simulink model "AUV_Model"  (R2023a)
settings: Solver=VariableStepAuto  StartTime=0.0  StopTime=300  FixedStep=0.5  RelTol=1e-3
InitFcn:
  | mdlWks = get_param(gcs,'ModelWorkspace');
  | a = getVariable(mdlWks,'a');
  | b = getVariable(mdlWks,'b');
  | c = getVariable(mdlWks,'c');
StopFcn:
  | figure(2)
  | plot3(Position_Data(1,1),Position_Data(1,2),Position_Data(1,3),'r*')
  | hold on
  | plot3(Position_Data(:,1),Position_Data(:,2),Position_Data(:,3));
  | plot3(Position_Data(end,1),Position_Data(end,2),Position_Data(end,3),'g*');
  | grid on
  | legend('Start Point','Trajectory','End Point')
model workspace (MAT data in the model file):
  a = 0
  b = 1
  c = 1
undefined symbols (not defined in the file or in its folder): sigbuilder_block
libraries: sharedtransform x6, vrlib x6, dspfdesign x6, sim3dlib x3, slpidlib x3, simulink x2, shared6dof x1, aerolibasang x1, aerolibnav x1, sim3dphyssensorlib x1
(part 2 of 2)

== system AUV_Model/Plant and Environment Model/Propulsion Forces & Moments/Force and moments due to Thrust/Thrust to Propulsion  ==
  Thrust Inputs : Inport
  Demux : Demux  Outputs=5
  Moment computation : Subsystem
  Sum : Sum  Inputs=+++++
  Thrust Transformation : Subsystem
  Propulsion Force : Outport  VectorParamsAs1DForOutWhenUnconnected=off
  Propulsion Moment : Outport  Port=2  VectorParamsAs1DForOutWhenUnconnected=off
  wires:
  Demux/5 -> Moment computation/5(Pz)
  Demux/4 -> Moment computation/4(Py2)
  Demux/3 -> Moment computation/3(Py1)
  Demux/2 -> Moment computation/2(Px2)
  Demux/1 -> Moment computation/1(Px1)
  Thrust Transformation/3(Thrust Py1) -> Sum/3
  Moment computation/1(Moment) -> Propulsion Moment/1
  Thrust Transformation/4(Thrust Py2) -> Sum/4
  Thrust Transformation/5(Thrust Pz) -> Sum/5
  Sum/1 -> Propulsion Force/1
  Thrust Inputs/1 -> Thrust Transformation/1(Thrust Inputs), Demux/1
  Thrust Transformation/1(Thrust Px1) -> Sum/1
  Thrust Transformation/2(Thrust Px2) -> Sum/2

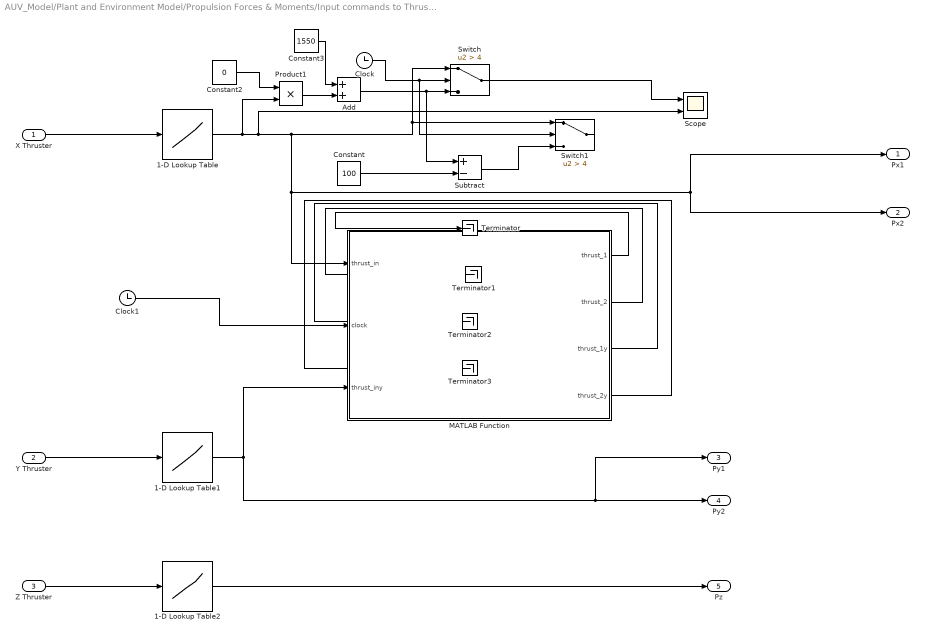
== system AUV_Model/Plant and Environment Model/Propulsion Forces & Moments/Input commands to Thrust/Input Commands to PWM ==
  X Thruster : Inport
  Y Thruster : Inport  Port=2
  Z Thruster : Inport  Port=3
  1-D Lookup Table : Lookup_n-D  NumberOfTableDimensions=1  BreakpointsForDimension1=[-1:0.01:1]  Table=1500 + 400 * ([-1:0.01:1])  InternalRulePriority=Speed  RndMeth=Simplest
  1-D Lookup Table1 : Lookup_n-D  NumberOfTableDimensions=1  BreakpointsForDimension1=[-1:0.01:1]  Table=1500 + 400 * ([-1:0.01:1])  InternalRulePriority=Speed  RndMeth=Simplest
  1-D Lookup Table2 : Lookup_n-D  NumberOfTableDimensions=1  BreakpointsForDimension1=[-1:0.01:1]  Table=1500 + 400 * ([-1:0.01:1])  InternalRulePriority=Speed  RndMeth=Simplest
  Add : Sum
  Clock : Clock
  Clock1 : Clock
  Constant : Constant  Value=100
  Constant2 : Constant  Value=0
  Constant3 : Constant  Value=1550
  MATLAB Function : MATLAB Function  TreatAsAtomicUnit=on
  Product1 : Product
  Scope : Scope  NumInputPorts=2
  Subtract : Sum  Inputs=+-
  Switch : Switch  Criteria=u2 > Threshold  Threshold=4  SaturateOnIntegerOverflow=off  InputSameDT=off
  Switch1 : Switch  Criteria=u2 > Threshold  Threshold=4  SaturateOnIntegerOverflow=off  InputSameDT=off
  Terminator{,1..3} (4 alike) : Terminator
  Px1 : Outport  VectorParamsAs1DForOutWhenUnconnected=off
  Px2 : Outport  Port=2  VectorParamsAs1DForOutWhenUnconnected=off
  Py1 : Outport  Port=3  VectorParamsAs1DForOutWhenUnconnected=off
  Py2 : Outport  Port=4  VectorParamsAs1DForOutWhenUnconnected=off
  Pz : Outport  Port=5  VectorParamsAs1DForOutWhenUnconnected=off
  wires:
  Y Thruster/1 -> 1-D Lookup Table1/1
  Z Thruster/1 -> 1-D Lookup Table2/1
  X Thruster/1 -> 1-D Lookup Table/1
  Constant/1 -> Subtract/2
  Clock/1 -> Switch1/2, Switch/2
  1-D Lookup Table2/1 -> Pz/1
  Constant2/1 -> Product1/1
  Product1/1 -> Add/2
  Constant3/1 -> Add/1
  Add/1 -> Subtract/1, Switch/3
  1-D Lookup Table/1 -> Scope/2, Px2/1, Px1/1, MATLAB Function/1(thrust_in), Switch1/1, Switch/1, Product1/2
  Subtract/1 -> Switch1/3
  Switch/1 -> Scope/1
  1-D Lookup Table1/1 -> MATLAB Function/3(thrust_iny), Py1/1, Py2/1
  Clock1/1 -> MATLAB Function/2(clock)
  MATLAB Function/1(thrust_1) -> Terminator/1
  MATLAB Function/2(thrust_2) -> Terminator1/1
  MATLAB Function/3(thrust_1y) -> Terminator2/1
  MATLAB Function/4(thrust_2y) -> Terminator3/1

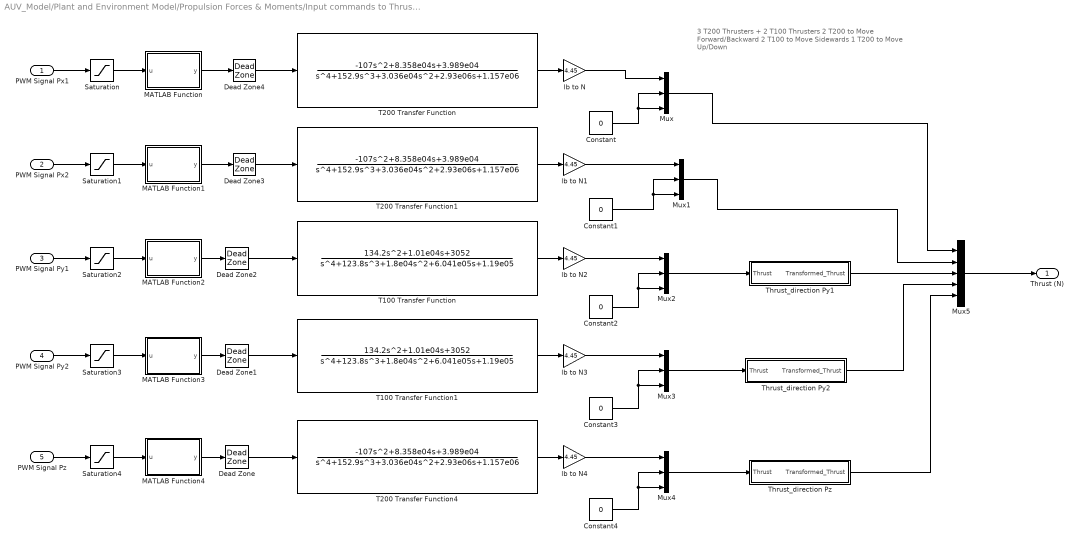
== system AUV_Model/Plant and Environment Model/Propulsion Forces & Moments/Input commands to Thrust/PWM Signals to Thrust  ==
  note: 3 T200 Thrusters + 2 T100 Thrusters
      |
      | 2 T200 to Move Forward/Backward
      | 2 T100 to Move Sidewards
      | 1 T200 to Move Up/Down
  PWM Signal Px1 : Inport
  PWM Signal Px2 : Inport  Port=2
  PWM Signal Py1 : Inport  Port=3
  PWM Signal Py2 : Inport  Port=4
  PWM Signal Pz : Inport  Port=5
  Constant{,1..4} (5 alike) : Constant  Value=0
  Dead Zone{,2..4} (4 alike) : DeadZone  LowerValue=-10  UpperValue=+10
  Dead Zone1 : DeadZone  LowerValue=-10  UpperValue=10
  MATLAB Function : MATLAB Function  TreatAsAtomicUnit=on
  MATLAB Function1 : MATLAB Function  TreatAsAtomicUnit=on
  MATLAB Function2 : MATLAB Function  TreatAsAtomicUnit=on
  MATLAB Function3 : MATLAB Function  TreatAsAtomicUnit=on
  MATLAB Function4 : MATLAB Function  TreatAsAtomicUnit=on
  Mux{,1..4} (5 alike) : Mux  Inputs=3
  Mux5 : Mux  Inputs=5
  Saturation{,1..4} (5 alike) : Saturate  UpperLimit=1900  LowerLimit=1100
  T100 Transfer Function : TransferFcn  Numerator="[134.2 1.01e04  3052]"  Denominator=[1 123.8 1.8e04 6.041e05 1.19e05]
  T100 Transfer Function1 : TransferFcn  Numerator="[134.2 1.01e04  3052]"  Denominator=[1 123.8 1.8e04 6.041e05 1.19e05]
  T200 Transfer Function : TransferFcn  Numerator="[-107  8.358e04  3.989e04]"  Denominator="[1 152.9  3.036e04  2.93e06  1.157e06]"
  T200 Transfer Function1 : TransferFcn  Numerator="[-107  8.358e04  3.989e04]"  Denominator="[1 152.9  3.036e04  2.93e06  1.157e06]"
  T200 Transfer Function4 : TransferFcn  Numerator="[-107  8.358e04  3.989e04]"  Denominator="[1 152.9  3.036e04  2.93e06  1.157e06]"
  Thrust_direction Py1 : Subsystem
  Thrust_direction Py2 : Subsystem
  Thrust_direction Pz : Subsystem
  lb to N{,1..4} (5 alike) : Gain  Gain=4.45
  Thrust (N) : Outport  VectorParamsAs1DForOutWhenUnconnected=off
  wires:
  Dead Zone4/1 -> T200 Transfer Function/1
  Dead Zone3/1 -> T200 Transfer Function1/1
  Dead Zone2/1 -> T100 Transfer Function/1
  Dead Zone1/1 -> T100 Transfer Function1/1
  Dead Zone/1 -> T200 Transfer Function4/1
  MATLAB Function4/1(y) -> Dead Zone/1
  MATLAB Function3/1(y) -> Dead Zone1/1
  MATLAB Function2/1(y) -> Dead Zone2/1
  MATLAB Function1/1(y) -> Dead Zone3/1
  Saturation3/1 -> MATLAB Function3/1(u)
  PWM Signal Py2/1 -> Saturation3/1
  Saturation4/1 -> MATLAB Function4/1(u)
  Saturation2/1 -> MATLAB Function2/1(u)
  Saturation1/1 -> MATLAB Function1/1(u)
  Saturation/1 -> MATLAB Function/1(u)
  MATLAB Function/1(y) -> Dead Zone4/1
  T100 Transfer Function1/1 -> lb to N3/1
  lb to N2/1 -> Mux2/1
  Mux4/1 -> Thrust_direction Pz/1(Thrust)
  Mux5/1 -> Thrust (N)/1
  Thrust_direction Pz/1("Transformed_Thrust ") -> Mux5/5
  lb to N/1 -> Mux/1
  Constant1/1 -> Mux1/2, Mux1/3
  T200 Transfer Function1/1 -> lb to N1/1
  Mux3/1 -> Thrust_direction Py2/1(Thrust)
  PWM Signal Pz/1 -> Saturation4/1
  PWM Signal Px1/1 -> Saturation/1
  Constant/1 -> Mux/2, Mux/3
  Thrust_direction Py2/1("Transformed_Thrust ") -> Mux5/4
  Thrust_direction Py1/1("Transformed_Thrust ") -> Mux5/3
  PWM Signal Py1/1 -> Saturation2/1
  lb to N1/1 -> Mux1/1
  lb to N4/1 -> Mux4/1
  Constant4/1 -> Mux4/2, Mux4/3
  T200 Transfer Function4/1 -> lb to N4/1
  T200 Transfer Function/1 -> lb to N/1
  Constant2/1 -> Mux2/2, Mux2/3
  Mux2/1 -> Thrust_direction Py1/1(Thrust)
  PWM Signal Px2/1 -> Saturation1/1
  Constant3/1 -> Mux3/2, Mux3/3
  lb to N3/1 -> Mux3/1
  T100 Transfer Function/1 -> lb to N2/1
  Mux1/1 -> Mux5/2
  Mux/1 -> Mux5/1

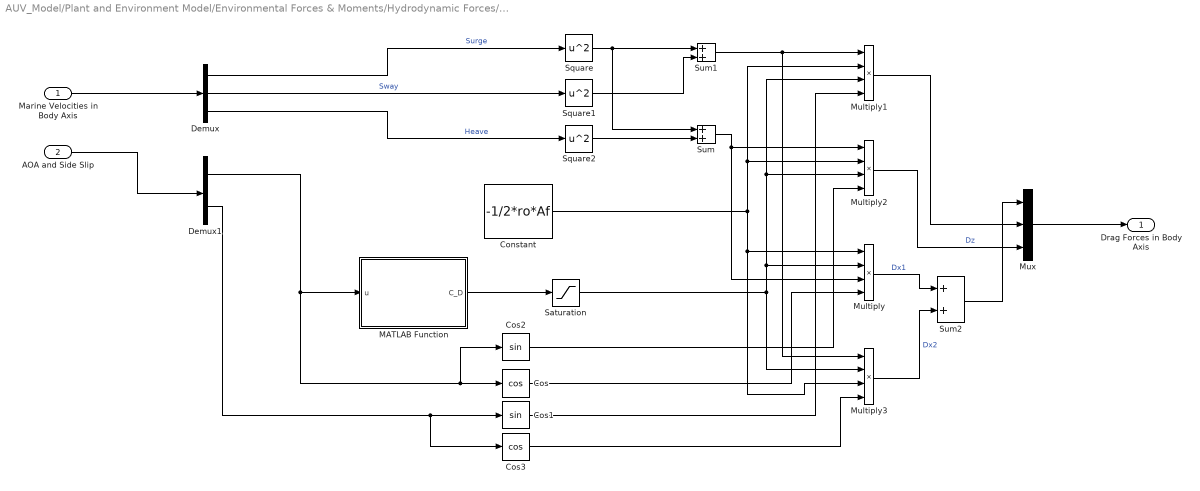
== system AUV_Model/Plant and Environment Model/Environmental Forces & Moments/Hydrodynamic Forces/Hydrodynamic Forces - Accurate/Force Exerted due to Drag (Body Axis) ==
  Marine Velocities in Body Axis : Inport
  AOA and Side Slip : Inport  Port=2
  Constant : Constant  Value=-1/2*ro*Af  mask{ro=1000, Af=0.001}
      mask prompts: ro "Density of Water"; Af "Submarine Frontal Area"
      mask DialogControl DescGroupVar Prompt: Input
      mask DialogControl DescTextVar Prompt: Enter the following values :
  Cos : Trigonometry  Operator=cos
  Cos1 : Trigonometry
  Cos2 : Trigonometry
  Cos3 : Trigonometry  Operator=cos
  Demux : Demux  Outputs=3
  Demux1 : Demux  Outputs=2
  MATLAB Function : MATLAB Function  TreatAsAtomicUnit=on
  Multiply{,1..3} (4 alike) : Product  Inputs=4
  Mux : Mux  Inputs=3
  Saturation : Saturate  UpperLimit=25  LowerLimit=-25
  Square : Math  Operator=square  SignedPower=on
  Square1 : Math  Operator=square  SignedPower=on
  Square2 : Math  Operator=square  SignedPower=on
  Sum : Sum
  Sum1 : Sum
  Sum2 : Sum
  Drag Forces in Body Axis : Outport  VectorParamsAs1DForOutWhenUnconnected=off
  wires:
  Saturation/1 -> Multiply/2, Multiply2/3, Multiply1/3, Multiply3/2
  Square1/1 -> Sum1/2
  Multiply1/1 -> Mux/2
  Sum2/1 -> Mux/1
  Cos3/1 -> Multiply3/4
  AOA and Side Slip/1 -> Demux1/1
  Marine Velocities in Body Axis/1 -> Demux/1
  Cos2/1 -> Multiply2/4
  Mux/1 -> Drag Forces in Body Axis/1
  Square2/1 -> Sum/2
  Demux1/2 -> Cos1/1, Cos3/1
  Demux1/1 -> MATLAB Function/1(u), Cos2/1, Cos/1
  MATLAB Function/1(C_D) -> Saturation/1
  Multiply2/1 -> Mux/3  "Dz"
  Cos/1 -> Multiply/4
  Demux/3 -> Square2/1  "Heave"
  Constant/1 -> Multiply2/2, Multiply1/2, Multiply/1, Multiply3/3
  Multiply3/1 -> Sum2/2  "Dx2"
  Sum/1 -> Multiply/3, Multiply2/1
  Demux/1 -> Square/1  "Surge"
  Multiply/1 -> Sum2/1  "Dx1"
  Sum1/1 -> Multiply1/1, Multiply3/1
  Cos1/1 -> Multiply1/4
  Demux/2 -> Square1/1  "Sway"
  Square/1 -> Sum1/1, Sum/1

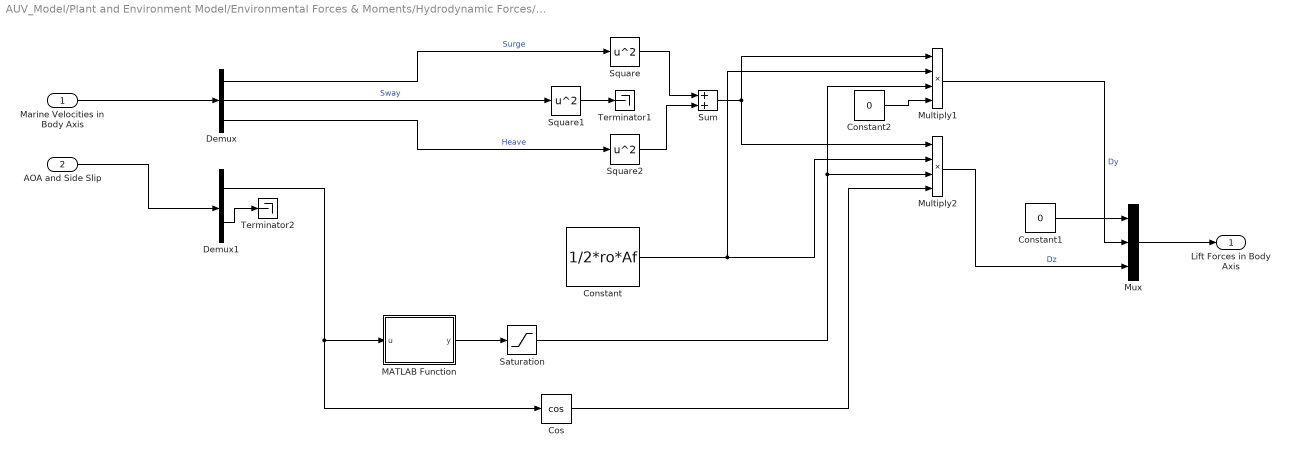
== system AUV_Model/Plant and Environment Model/Environmental Forces & Moments/Hydrodynamic Forces/Hydrodynamic Forces - Accurate/Force Exerted due to Lift (Body Axis) ==
  Marine Velocities in Body Axis : Inport
  AOA and Side Slip : Inport  Port=2
  Constant : Constant  Value=1/2*ro*Af  mask{ro=1000, Af=0.001}
      mask prompts: ro "Density of Water"; Af "Submarine Frontal Area"
      mask DialogControl DescGroupVar Prompt: Input
      mask DialogControl DescTextVar Prompt: Enter the following values :
  Constant1 : Constant  Value=0
  Constant2 : Constant  Value=0
  Cos : Trigonometry  Operator=cos
  Demux : Demux  Outputs=3
  Demux1 : Demux  Outputs=2
  MATLAB Function : MATLAB Function  TreatAsAtomicUnit=on
  Multiply1 : Product  Inputs=4
  Multiply2 : Product  Inputs=4
  Mux : Mux  Inputs=3
  Saturation : Saturate  UpperLimit=25  LowerLimit=-25
  Square : Math  Operator=square  SignedPower=on
  Square1 : Math  Operator=square  SignedPower=on
  Square2 : Math  Operator=square  SignedPower=on
  Sum : Sum
  Terminator1 : Terminator
  Terminator2 : Terminator
  Lift Forces in Body Axis : Outport  VectorParamsAs1DForOutWhenUnconnected=off
  wires:
  Saturation/1 -> Multiply2/3, Multiply1/3
  Constant2/1 -> Multiply1/4
  Multiply2/1 -> Mux/3  "Dz"
  Constant1/1 -> Mux/1
  Cos/1 -> Multiply2/4
  Square/1 -> Sum/1
  Demux/2 -> Square1/1  "Sway"
  Demux/1 -> Square/1  "Surge"
  Sum/1 -> Multiply1/1, Multiply2/1
  Constant/1 -> Multiply1/2, Multiply2/2
  Multiply1/1 -> Mux/2  "Dy"
  Demux/3 -> Square2/1  "Heave"
  MATLAB Function/1(y) -> Saturation/1
  Demux1/1 -> MATLAB Function/1(u), Cos/1
  Square2/1 -> Sum/2
  Mux/1 -> Lift Forces in Body Axis/1
  Marine Velocities in Body Axis/1 -> Demux/1
  AOA and Side Slip/1 -> Demux1/1
  Square1/1 -> Terminator1/1
  Demux1/2 -> Terminator2/1

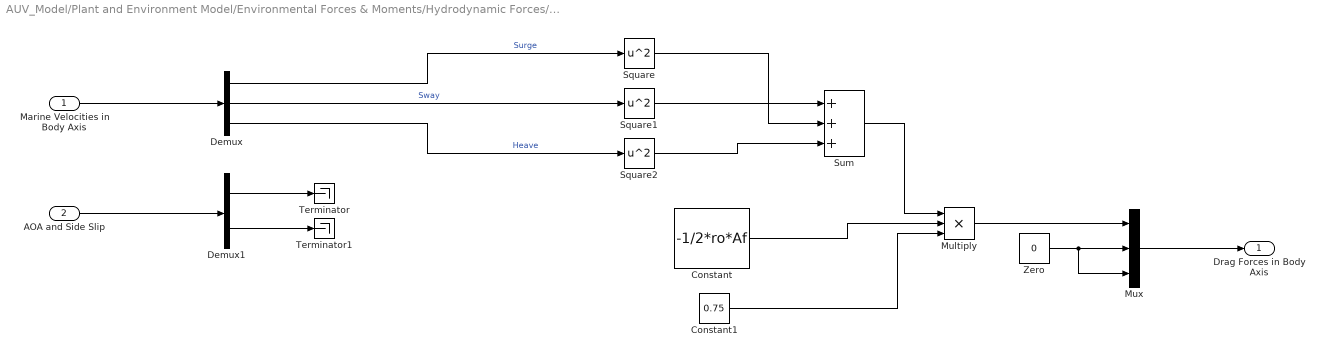
== system AUV_Model/Plant and Environment Model/Environmental Forces & Moments/Hydrodynamic Forces/Hydrodynamic Forces - Basic/Force Exerted due to Drag (Body Axis) ==
  Marine Velocities in Body Axis : Inport
  AOA and Side Slip : Inport  Port=2
  Constant : Constant  Value=-1/2*ro*Af  mask{ro=1000, Af=0.001}
      mask prompts: ro "Density of Water"; Af "Submarine Frontal Area"
      mask DialogControl DescGroupVar Prompt: Input
      mask DialogControl DescTextVar Prompt: Enter the following values :
  Constant1 : Constant  Value=0.75
  Demux : Demux  Outputs=3
  Demux1 : Demux  Outputs=2
  Multiply : Product  Inputs=3
  Mux : Mux  Inputs=3
  Square : Math  Operator=square  SignedPower=on
  Square1 : Math  Operator=square  SignedPower=on
  Square2 : Math  Operator=square  SignedPower=on
  Sum : Sum  Inputs=+++
  Terminator : Terminator
  Terminator1 : Terminator
  Zero : Constant  Value=0  OutDataTypeStr=Inherit: Inherit via back propagation
  Drag Forces in Body Axis : Outport  VectorParamsAs1DForOutWhenUnconnected=off
  wires:
  AOA and Side Slip/1 -> Demux1/1
  Marine Velocities in Body Axis/1 -> Demux/1
  Mux/1 -> Drag Forces in Body Axis/1
  Square2/1 -> Sum/3
  Demux/3 -> Square2/1  "Heave"
  Sum/1 -> Multiply/1
  Demux/1 -> Square/1  "Surge"
  Demux/2 -> Square1/1  "Sway"
  Square/1 -> Sum/2
  Square1/1 -> Sum/1
  Demux1/1 -> Terminator/1
  Demux1/2 -> Terminator1/1
  Constant/1 -> Multiply/2
  Constant1/1 -> Multiply/3
  Multiply/1 -> Mux/1
  Zero/1 -> Mux/3, Mux/2

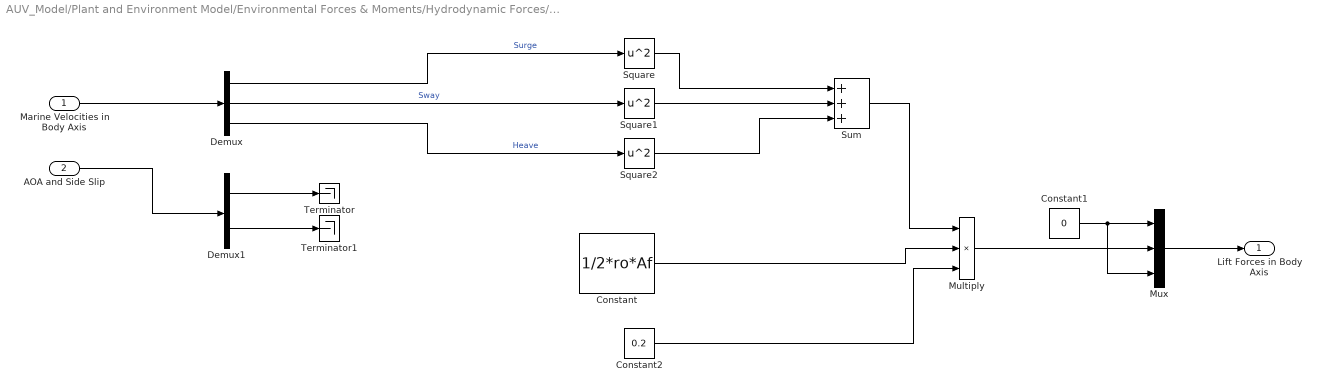
== system AUV_Model/Plant and Environment Model/Environmental Forces & Moments/Hydrodynamic Forces/Hydrodynamic Forces - Basic/Force Exerted due to Lift (Body Axis) ==
  Marine Velocities in Body Axis : Inport
  AOA and Side Slip : Inport  Port=2
  Constant : Constant  Value=1/2*ro*Af  mask{ro=1000, Af=0.001}
      mask prompts: ro "Density of Water"; Af "Submarine Frontal Area"
      mask DialogControl DescGroupVar Prompt: Input
      mask DialogControl DescTextVar Prompt: Enter the following values :
  Constant1 : Constant  Value=0
  Constant2 : Constant  Value=0.2
  Demux : Demux  Outputs=3
  Demux1 : Demux  Outputs=2
  Multiply : Product  Inputs=3
  Mux : Mux  Inputs=3
  Square : Math  Operator=square  SignedPower=on
  Square1 : Math  Operator=square  SignedPower=on
  Square2 : Math  Operator=square  SignedPower=on
  Sum : Sum  Inputs=+++
  Terminator : Terminator
  Terminator1 : Terminator
  Lift Forces in Body Axis : Outport  VectorParamsAs1DForOutWhenUnconnected=off
  wires:
  Constant1/1 -> Mux/3, Mux/1
  Square/1 -> Sum/1
  Demux/2 -> Square1/1  "Sway"
  Demux/1 -> Square/1  "Surge"
  Demux/3 -> Square2/1  "Heave"
  Square2/1 -> Sum/3
  Mux/1 -> Lift Forces in Body Axis/1
  Marine Velocities in Body Axis/1 -> Demux/1
  AOA and Side Slip/1 -> Demux1/1
  Square1/1 -> Sum/2
  Sum/1 -> Multiply/1
  Constant/1 -> Multiply/2
  Constant2/1 -> Multiply/3
  Multiply/1 -> Mux/2
  Demux1/1 -> Terminator/1
  Demux1/2 -> Terminator1/1

== system AUV_Model/Plant and Environment Model/Environmental Forces & Moments/Hydrostatic Forces/Environment Model/3D Rotate Drag ==
  Force : Inport
  "Roll, Pitch, Yaw" : Inport  Port=2
  Gain : Gain
  Matrix Multiply : Product  Multiplication=Matrix(*)
  Rotation Angles to Direction Cosine Matrix : sharedtransform/Rotation Angles to Direction Cosine Matrix  rotationOrder=XYZ  aMode=aMode
  Transpose : Math  Operator=transpose  SignedPower=on
  "Transformed_Force " : Outport  VectorParamsAs1DForOutWhenUnconnected=off
  wires:
  Matrix Multiply/1 -> "Transformed_Force "/1
  Rotation Angles to Direction Cosine Matrix/1 -> Transpose/1
  Force/1 -> Matrix Multiply/2
  "Roll, Pitch, Yaw"/1 -> Gain/1
  Transpose/1 -> Matrix Multiply/1
  Gain/1 -> Rotation Angles to Direction Cosine Matrix/1

== system AUV_Model/Plant and Environment Model/Propulsion Forces & Moments/Force and moments due to Thrust/Thrust to Propulsion /Moment computation ==
  Px1 : Inport
  Px2 : Inport  Port=2
  Py1 : Inport  Port=3
  Py2 : Inport  Port=4
  Pz : Inport  Port=5
  Moment Px1 : Subsystem  mask{a=0, b=-0.2, c=0}
      mask prompts: a "X Coordinate of Thruster from Center of Buoyancy"; b "Y Coordinate of Thruster from Center of Buoyancy"; c "Z Coordinate of Thruster from Center of Buoyancy"
      mask DialogControl DescTextVar Prompt: Enter Thruster Position w.r.t Center of Buoyancy
  Moment Px2 : Subsystem  mask{a=0, b=0.2, c=0}
      mask prompts: a "X Coordinate of Thruster from Center of Buoyancy"; b "Y Coordinate of Thruster from Center of Buoyancy"; c "Z Coordinate of Thruster from Center of Buoyancy"
      mask DialogControl DescTextVar Prompt: Enter Thruster Position w.r.t Center of Buoyancy
  Moment Py1 : Subsystem  mask{a=.2, b=0, c=0}
      mask prompts: a "X Coordinate of Thruster from Center of Buoyancy"; b "Y Coordinate of Thruster from Center of Buoyancy"; c "Z Coordinate of Thruster from Center of Buoyancy"
      mask DialogControl DescTextVar Prompt: Enter Thruster Position w.r.t Center of Buoyancy
  Moment Py2 : Subsystem  mask{a=-0.2, b=0, c=0}
      mask prompts: a "X Coordinate of Thruster from Center of Buoyancy"; b "Y Coordinate of Thruster from Center of Buoyancy"; c "Z Coordinate of Thruster from Center of Buoyancy"
      mask DialogControl DescTextVar Prompt: Enter Thruster Position w.r.t Center of Buoyancy
  Moment Pz : Subsystem  mask{a=0, b=0, c=0}
      mask prompts: a "X Coordinate of Thruster from Center of Buoyancy"; b "Y Coordinate of Thruster from Center of Buoyancy"; c "Z Coordinate of Thruster from Center of Buoyancy"
      mask DialogControl DescTextVar Prompt: Enter Thruster Position w.r.t Center of Buoyancy
  Scope : Scope
  Scope1 : Scope
  Sum1 : Sum  Inputs=+++++
  Moment : Outport  VectorParamsAs1DForOutWhenUnconnected=off
  wires:
  Py2/1 -> Moment Py2/1(Thrust)
  Px1/1 -> Moment Px1/1(Thrust)
  Py1/1 -> Moment Py1/1(Thrust)
  Moment Px1/1(Moment) -> Scope/1, Sum1/1
  Moment Px2/1(Moment) -> Scope1/1, Sum1/2
  Moment Pz/1(Moment) -> Sum1/5
  Moment Py2/1(Moment) -> Sum1/4
  Pz/1 -> Moment Pz/1(Thrust)
  Moment Py1/1(Moment) -> Sum1/3
  Sum1/1 -> Moment/1
  Px2/1 -> Moment Px2/1(Thrust)

== system AUV_Model/Plant and Environment Model/Propulsion Forces & Moments/Force and moments due to Thrust/Thrust to Propulsion /Thrust Transformation ==
  Thrust Inputs : Inport
  Demux1 : Demux  Outputs=5
  Thrust Px1 : Outport  VectorParamsAs1DForOutWhenUnconnected=off
  Thrust Px2 : Outport  Port=2  VectorParamsAs1DForOutWhenUnconnected=off
  Thrust Py1 : Outport  Port=3  VectorParamsAs1DForOutWhenUnconnected=off
  Thrust Py2 : Outport  Port=4  VectorParamsAs1DForOutWhenUnconnected=off
  Thrust Pz : Outport  Port=5  VectorParamsAs1DForOutWhenUnconnected=off
  wires:
  Demux1/4 -> Thrust Py2/1
  Demux1/5 -> Thrust Pz/1
  Thrust Inputs/1 -> Demux1/1
  Demux1/1 -> Thrust Px1/1
  Demux1/2 -> Thrust Px2/1
  Demux1/3 -> Thrust Py1/1

== system AUV_Model/Plant and Environment Model/Propulsion Forces & Moments/Input commands to Thrust/PWM Signals to Thrust /Thrust_direction Py1 ==
  Thrust : Inport
  Constant : Constant  Value=0
  Constant1 : Constant  Value=0
  Constant2 : Constant  Value=pi/2
  Matrix Multiply : Product  Multiplication=Matrix(*)
  Mux : Mux  Inputs=3
  Rotation Angles to Direction Cosine Matrix : sharedtransform/Rotation Angles to Direction Cosine Matrix  rotationOrder=XYZ  aMode=aMode
  Transpose : Math  Operator=transpose  SignedPower=on
  "Transformed_Thrust " : Outport  VectorParamsAs1DForOutWhenUnconnected=off
  wires:
  Matrix Multiply/1 -> "Transformed_Thrust "/1
  Mux/1 -> Rotation Angles to Direction Cosine Matrix/1
  Rotation Angles to Direction Cosine Matrix/1 -> Transpose/1
  Constant1/1 -> Mux/2
  Thrust/1 -> Matrix Multiply/2
  Constant/1 -> Mux/1
  Transpose/1 -> Matrix Multiply/1
  Constant2/1 -> Mux/3

== system AUV_Model/Plant and Environment Model/Propulsion Forces & Moments/Input commands to Thrust/PWM Signals to Thrust /Thrust_direction Py2 ==
  Thrust : Inport
  Constant : Constant  Value=0
  Constant1 : Constant  Value=0
  Constant2 : Constant  Value=pi/2
  Matrix Multiply : Product  Multiplication=Matrix(*)
  Mux : Mux  Inputs=3
  Rotation Angles to Direction Cosine Matrix : sharedtransform/Rotation Angles to Direction Cosine Matrix  rotationOrder=XYZ  aMode=aMode
  Transpose : Math  Operator=transpose  SignedPower=on
  "Transformed_Thrust " : Outport  VectorParamsAs1DForOutWhenUnconnected=off
  wires:
  Matrix Multiply/1 -> "Transformed_Thrust "/1
  Mux/1 -> Rotation Angles to Direction Cosine Matrix/1
  Rotation Angles to Direction Cosine Matrix/1 -> Transpose/1
  Constant1/1 -> Mux/2
  Thrust/1 -> Matrix Multiply/2
  Constant/1 -> Mux/1
  Transpose/1 -> Matrix Multiply/1
  Constant2/1 -> Mux/3

== system AUV_Model/Plant and Environment Model/Propulsion Forces & Moments/Input commands to Thrust/PWM Signals to Thrust /Thrust_direction Pz ==
  Thrust : Inport
  Constant : Constant  Value=0
  Constant1 : Constant  Value=pi/2
  Constant2 : Constant  Value=0
  Matrix Multiply : Product  Multiplication=Matrix(*)
  Mux : Mux  Inputs=3
  Rotation Angles to Direction Cosine Matrix : sharedtransform/Rotation Angles to Direction Cosine Matrix  rotationOrder=ZYX  aMode=aMode
  Transpose : Math  Operator=transpose  SignedPower=on
  "Transformed_Thrust " : Outport  VectorParamsAs1DForOutWhenUnconnected=off
  wires:
  Matrix Multiply/1 -> "Transformed_Thrust "/1
  Mux/1 -> Rotation Angles to Direction Cosine Matrix/1
  Rotation Angles to Direction Cosine Matrix/1 -> Transpose/1
  Constant1/1 -> Mux/2
  Thrust/1 -> Matrix Multiply/2
  Constant/1 -> Mux/1
  Transpose/1 -> Matrix Multiply/1
  Constant2/1 -> Mux/3

== system AUV_Model/Plant and Environment Model/Propulsion Forces & Moments/Force and moments due to Thrust/Thrust to Propulsion /Moment computation/Moment Px1 ==
  Thrust : Inport
  Constant : Constant  Value=[a;b;c]
  Cross Product : vrlib/Utilities/Cross Product
  Moment : Outport  VectorParamsAs1DForOutWhenUnconnected=off
  wires:
  Cross Product/1 -> Moment/1
  Thrust/1 -> Cross Product/2
  Constant/1 -> Cross Product/1

== system AUV_Model/Plant and Environment Model/Propulsion Forces & Moments/Force and moments due to Thrust/Thrust to Propulsion /Moment computation/Moment Px2 ==
  Thrust : Inport
  Constant : Constant  Value=[a;b;c]
  Cross Product : vrlib/Utilities/Cross Product
  Moment : Outport  VectorParamsAs1DForOutWhenUnconnected=off
  wires:
  Constant/1 -> Cross Product/1
  Thrust/1 -> Cross Product/2
  Cross Product/1 -> Moment/1

== system AUV_Model/Plant and Environment Model/Propulsion Forces & Moments/Force and moments due to Thrust/Thrust to Propulsion /Moment computation/Moment Py1 ==
  Thrust : Inport
  Constant : Constant  Value=[a;b;c]
  Cross Product : vrlib/Utilities/Cross Product
  Moment : Outport  VectorParamsAs1DForOutWhenUnconnected=off
  wires:
  Cross Product/1 -> Moment/1
  Thrust/1 -> Cross Product/2
  Constant/1 -> Cross Product/1

== system AUV_Model/Plant and Environment Model/Propulsion Forces & Moments/Force and moments due to Thrust/Thrust to Propulsion /Moment computation/Moment Py2 ==
  Thrust : Inport
  Constant : Constant  Value=[a;b;c]
  Cross Product : vrlib/Utilities/Cross Product
  Moment : Outport  VectorParamsAs1DForOutWhenUnconnected=off
  wires:
  Constant/1 -> Cross Product/1
  Thrust/1 -> Cross Product/2
  Cross Product/1 -> Moment/1

== system AUV_Model/Plant and Environment Model/Propulsion Forces & Moments/Force and moments due to Thrust/Thrust to Propulsion /Moment computation/Moment Pz ==
  Thrust : Inport
  Constant : Constant  Value=[a;b;c]
  Cross Product : vrlib/Utilities/Cross Product
  Moment : Outport  VectorParamsAs1DForOutWhenUnconnected=off
  wires:
  Cross Product/1 -> Moment/1
  Thrust/1 -> Cross Product/2
  Constant/1 -> Cross Product/1

== matlab function AUV_Model/Plant and Environment Model/Propulsion Forces & Moments/Input commands to Thrust/Input Commands to PWM/MATLAB Function ==
  data: thrust_in input; thrust_1 output; clock input; thrust_2 output; thrust_1y output; thrust_2y output; thrust_iny input
function [thrust_1, thrust_2,thrust_1y, thrust_2y]= turn_logic(thrust_in, clock, thrust_iny)

if clock<4
    thrust_1=1450;
    thrust_2=1550;
elseif clock > 4 && clock < 8
    thrust_1=1550;
    thrust_2=1450;
elseif clock >8
    thrust_1=thrust_in;
    thrust_2=thrust_in;
else
    thrust_1=1500;
    thrust_2=1500;
end


if clock >8
    thrust_1y=1500;
    thrust_2y=1500;
else
    thrust_1y=thrust_iny;
    thrust_2y=thrust_iny;
end

== matlab function AUV_Model/LiDAR Test Data/Lidar control ==
  data: point_cloud input; idle_control output; clock input; state_o output
function [idle_control,state_o]= lidar_control(point_cloud, clock)

%Params
%%%%%%%%%%%%%%%%%%%%%%%%%%%%%%%%%%%%%%%%
num_points_x=0;
num_points_z=0;
crack_width=5;
crack_depth=3;
scan_period=3;
%%%%%%%%%%%%%%%%%%%%%%%%%%%%%%%%%%%%%%%%


%States of Robot
%%%%%%%%%%%%%%%%%%%%%%%%%%%%%%%%%%%%%%%%
persistent state;
moving = 0; %Moving along the structure
scanning = 1; %Stop to scan
crack_detected=2; %Investigating crack
%%%%%%%%%%%%%%%%%%%%%%%%%%%%%%%%%%%%%%%%


%Other persistent vars
%%%%%%%%%%%%%%%%%%%%%%%%%%%%%%%%%%%%%%%%
persistent idle_ref;
%%%%%%%%%%%%%%%%%%%%%%%%%%%%%%%%%%%%%%%%


%State Initalization
%%%%%%%%%%%%%%%%%%%%%%%%%%%%%%%%%%%%%%%%
if isempty(state)
    state=0;
    idle_ref=1;
end
%%%%%%%%%%%%%%%%%%%%%%%%%%%%%%%%%%%%%%%%


%Moving State
%%%%%%%%%%%%%%%%%%%%%%%%%%%%%%%%%%%%%%%%
if state==moving
    
    idle_ref=1;

    %Perform scan every 5 seconds
    if mod(clock,scan_period)==0 && clock >0
        state=scanning;
    end

end
%%%%%%%%%%%%%%%%%%%%%%%%%%%%%%%%%%%%%%%%


%Scanning State
%%%%%%%%%%%%%%%%%%%%%%%%%%%%%%%%%%%%%%%%
if state == scanning

    idle_ref=0; %stop the robot

    pcloud=point_cloud; %get point cloud data

    %depth coordinates of dam surface
    ycoords=pcloud(:,:,2);

    %set the average depth to 0
    avg=mean(ycoords(:));
    ycoords=ycoords-avg;

    %Searching for vertical cracks
    for i=1:size(ycoords,1)

        %look at individual row
        row = ycoords(i,:);

        count=0; %counter var

        %scan the row
        for j=1:size(row,2)

            %Look for consecutive values well above the average depth
            if row(j)>crack_depth
                count= count+1;
                if count > crack_width
                    state=crack_detected;
                end
            else
                count=0;
            end

        end
    end


    
    %Searching for horizontal cracks
    for i=1:size(ycoords,2)

        %Look at individual column
        col = ycoords(:,i);

        count=0; %counter var

        %scan column
        for j=1:size(col,1)
            if col(j)>crack_depth
                count= count+1;

                %If multiple values above threshold are found, a crack
                %has been found
                if count > crack_width
                    state=crack_detected;
                end
            else
                count=0;
            end
        end
    end


    %If no crack was detected, go back to moving
    if state==scanning
        state=moving;
    end

end
%%%%%%%%%%%%%%%%%%%%%%%%%%%%%%%%%%%%%%%%

%Crack Detected State
%%%%%%%%%%%%%%%%%%%%%%%%%%%%%%%%%%%%%%%%
if state == crack_detected

    idle_ref=0; %fixate

    %Todo: action when crack is detected?
end
%%%%%%%%%%%%%%%%%%%%%%%%%%%%%%%%%%%%%%%%


%Sync outputs
idle_control=idle_ref;
state_o=state;

== matlab function AUV_Model/Plant and Environment Model/Dynamics solver/Turn Control/MATLAB Function1 ==
  data: actual_angle input; angle output; target_angle input
function angle = turn_controller(actual_angle, target_angle)

if isempty(actual_angle)
    angle=0;
end


if (actual_angle==target_angle)==false
    angle = actual_angle+(target_angle-actual_angle)*.01;
else
    angle=actual_angle;
end


end

== matlab function AUV_Model/LiDAR Test Data/MATLAB Function ==
  data: pcloud output; x input; y input; z input
function pcloud = fcn(x,y,z)

persistent array

if isempty(array)
    array=rand(1000,1000,3);
    for i=1:1000
        for j=1:1000
            array(i,j,1)=i/100;
            array(i,j,3)=j/100;
            if i >400 && i <600
                array(i,j,2)=4+rand;
            end
        end
    end
end



pcloud=array;

== matlab function AUV_Model/LiDAR Test Data/MATLAB Function1 ==
  data: pcloud output; x input; y input; z input
function pcloud = fcn(x,y,z)

persistent array

if isempty(array)
    array=rand(1000,1000,3);
    for i=1:1000
        for j=1:1000
            array(i,j,1)=i/100;
            array(i,j,3)=j/100;
        end
    end
end



pcloud=array;

== matlab function AUV_Model/Plant and Environment Model/Environmental Forces & Moments/Hydrodynamic Forces/Hydrodynamic Forces - Accurate/Force Exerted due to Drag (Body Axis)/MATLAB Function ==
  data: u input; C_D output
function C_D = Calculate_Drag_Coeff(u)
if u>pi/2
    u = u-pi;
elseif u < -pi/2
    u = u + pi;
end
C_D = 5.25*(u.^2) - 0.315 * (u) + 0.732;

== matlab function AUV_Model/Plant and Environment Model/Environmental Forces & Moments/Hydrodynamic Forces/Hydrodynamic Forces - Accurate/Force Exerted due to Lift (Body Axis)/MATLAB Function ==
  data: u input; y output
function y = fcn(u)
if u>pi/2
    u = u-pi;
elseif u < -pi/2
    u = u + pi;
end

y = 1 * (u) + 0;

== matlab function AUV_Model/Plant and Environment Model/Propulsion Forces & Moments/Input commands to Thrust/PWM Signals to Thrust /MATLAB Function ==
  data: u input; y output
function y = Normalize(u)
y = (u-1500)*150/400;

== matlab function AUV_Model/Plant and Environment Model/Propulsion Forces & Moments/Input commands to Thrust/PWM Signals to Thrust /MATLAB Function1 ==
  data: u input; y output
function y = Normalize(u)
y = (u-1500)*150/400;

== matlab function AUV_Model/Plant and Environment Model/Propulsion Forces & Moments/Input commands to Thrust/PWM Signals to Thrust /MATLAB Function2 ==
  data: u input; y output
function y = Normalize(u)
y = (u-1500)*150/400;

== matlab function AUV_Model/Plant and Environment Model/Propulsion Forces & Moments/Input commands to Thrust/PWM Signals to Thrust /MATLAB Function3 ==
  data: u input; y output
function y = Normalize(u)
y = (u-1500)*150/400;

== matlab function AUV_Model/Plant and Environment Model/Propulsion Forces & Moments/Input commands to Thrust/PWM Signals to Thrust /MATLAB Function4 ==
  data: u input; y output
function y = Normalize(u)
y = (u-1500)*150/400;

== matlab function AUV_Model/Plant and Environment Model/Dynamics solver/Post-Processing/MATLAB Function ==
  data: Position input; srf_in input
function Visualize(Position, srf_in)

    coder.extrinsic('setax'); 
    setax(Position, srf_in);  

end

== matlab function AUV_Model/Translational Reference/Dam Scanner Logic/MATLAB Function ==
  data: depth input; x output; length input; pass_height input; act_x input; act_y input; act_z input; y output; z output
function [x, y, z]= dam_scanner(depth, length, pass_height, act_x, act_y, act_z)

%Init reference params
persistent ref_x;
persistent ref_y;
persistent ref_z;

%4 step types
persistent step_type;

if isempty(ref_x)
    ref_x=0;
    ref_y=0;
    ref_z=0;
    step_type=0;
end


    % If the robot has reached its reference position, update
if(abs(act_x-ref_x)<2 && abs(act_y-ref_y)<2 && abs(act_z-ref_z)<2)
    
    if ref_z==depth
        step_type=4;
        ref_x=0;
        ref_y=0;
        ref_z=0;
    end

        %Cross away
    if(step_type==0)
        ref_y = ref_y + length;
        step_type=1;

        
        %Dive
    elseif(step_type==1)
        ref_z = ref_z - pass_height;
        step_type=2;
 
        
        %Cross back
    elseif(step_type==2)
        ref_y = ref_y - length;
        step_type=3;
    
        
        %Dive
    elseif(step_type==3)
        ref_z = ref_z - pass_height;
        step_type=0;
    end
end

x=ref_x;
y=ref_y;
z=ref_z;

end

== matlab function AUV_Model/Translational Reference/Pillar Scanner Logic/MATLAB Function ==
  data: depth input; diameter input; x output; pass_height input; act_x input; act_y input; act_z input; y output; z output; target_angle output
function [x, y, z, target_angle]= pillar_scanner(depth,diameter, pass_height, act_x, act_y, act_z)

%Init reference params
persistent ref_x;
persistent ref_y;
persistent ref_z;
persistent ref_target_angle;

%4 step types
persistent step_type;

if isempty(ref_x)
    ref_x=0;
    ref_y=0;
    ref_z=0;
    step_type=0;
    ref_target_angle=-pi()/4;
end


    % If the robot has reached its reference position, update
if(abs(act_x-ref_x)<4 && abs(act_y-ref_y)<4 && abs(act_z-ref_z)<4)
    
    if ref_z==-depth
        step_type=5;
        ref_x=0;
        ref_y=0;
        ref_z=0;
    end

    %Go to side 1
    if(step_type==0)
        ref_y = ref_y + (diameter+4)/2;
        step_type=1;
        ref_target_angle = ref_target_angle+ pi()/4;
  

        %Go to corner 2
    elseif(step_type==1)
        ref_y = ref_y + (diameter+4)/2;
        step_type=2;
        ref_target_angle = ref_target_angle+ pi()/4;
    
    %Go to side 2
    elseif(step_type==2)
        ref_x = ref_x + (diameter+4)/2;
        step_type=3;
        ref_target_angle = ref_target_angle+ pi()/4;
        
        %Go to corner 3
    elseif(step_type==3)
        ref_x = ref_x + (diameter+4)/2;
        step_type=4;
        ref_target_angle = ref_target_angle+ pi()/4;
    
    %Go to side 3
    elseif(step_type==4)
        ref_y = ref_y - (diameter+4)/2;
        step_type=5;
        ref_target_angle = ref_target_angle+ pi()/4;
        
        %Go to corner 4
    elseif(step_type==5)
        ref_y = ref_y - (diameter+4)/2;
        step_type=6;
        ref_target_angle = ref_target_angle+ pi()/4;
    
    %Go to side 4
    elseif(step_type==6)
        ref_x = ref_x - (diameter+4)/2;
        step_type=7;
        ref_target_angle = ref_target_angle+ pi()/4;
        
        %Go to corner 1
    elseif(step_type==7)
        ref_x = ref_x - (diameter+4)/2;
        step_type=8;
        ref_target_angle = ref_target_angle+ pi()/4;

        %Dive
    elseif(step_type==8)
        ref_z = ref_z - pass_height;
        step_type=0;
    end

end

x=ref_x;
y=ref_y;
z=ref_z;
target_angle=ref_target_angle;

end
